simulink library "LPVBlockLibrary"  (R2014b)
settings: Solver=ode45  StartTime=0.0  StopTime=10.0  RelTol=1e-3
values from neighbouring files (symbols this model uses):
  ABMat = {Mab11, Mab12, Mab21, Mab22}    [lpvblkinit.m]
  CDMat = {Mcd11, Mcd12, Mcd21, Mcd22}    [lpvblkinit.m]
  dIVData = nan    [lpvblkinit.m]
  IVData = cell(numel(loc),1)    [lpvblkinit.m]
  LIVData = LIVData(loc)    [lpvblkinit.m]
  niv = numel(plist)    [lpvblkinit.m]
  nU = szS(2)    [lpvblkinit.m]
undefined symbols (not defined in the file or in its folder): x0
undefined symbols (not defined in the file): sys
libraries: LPVBlockLibrary x1
settings Model: Creator=musyn  LastModifiedBy=Arnar

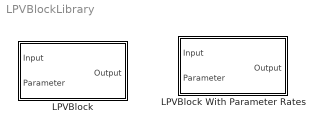
== system LPVBlockLibrary ==
  LPVBlock : Subsystem  mask{sys=sys, plist={'rho'}, x0=0}
      mask prompts: sys "System"; plist "ParameterVectorInputList (cell)"; x0 "Initial Condition"
      mask init:
      | [nU,ABMat,CDMat,IVData,dIVData,niv,LIVData] = ...
      |     lpvblkinit(sys,plist);
  LPVBlock With Parameter Rates : Subsystem  mask{sys=sys, plist={'rho'}, x0=x0, ratetc={'rho' 0.01}}
      mask prompts: sys "System"; plist "ParameterVectorInputList (cell)"; x0 "Initial Condition"; ratetc "Parameter Rate Time Constants"
      mask help:
      | Parameter Rate Time Constants:
      | N-by-2 cell array with each row being
      |    { char, time constant}.
      | The char specifies the parameter to be differentiated, e.g. 'rho'.
      | This parameter value will be approximately differentiated using
      | a high pass filter with the specified time constant.  The parameter
      | derivative must be an independent variable of the input PSS
      | specified in the form [char 'Dot'], e.g. 'rhoDot'.
      mask init:
      | if size(ratetc,2)~=2
      |     error('Parameter Rate Time Constants must be an N-by-2 cell array');
      | end
      | nrate = size(ratetc,1);
      | prate = ratetc(:,1);
      | nplist = length(plist);
      | 
      | [tfidx,prateidx] = ismember(prate,plist);
      | if all(tfidx)
      |     for i=1:nrate
      |         prate{i} = [prate{i} 'Dot'];
      |     end    
      |     pALL = [plist(:); prate(:)];
      | else
      |     % TODO PJS 5/28/2011: Improve error messages
      |     error('Parameters listed in rate time constants must be a subset of Parameter list');
      | end
      | 
      | % Convert to state space form
      | %   G(s) = s/(tau*s+1) = 1/tau
      | %
      | %   tau dx/dt +x = u
      | % --> dx/dt = -1/tau *x + 1/tau *u
      | tc = cell2mat(ratetc(:,2));
      | Ahp = diag( -1./tc );
      | Bhp = diag( -1./tc );
      | Chp = diag(  1./tc );
      | Dhp = diag(  1./tc );
      | 
      | % TODO PJS 5/28/2011: How should filter initial
      | % condition be handled?
      | xhp0 = zeros(nrate,1);

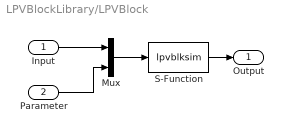
== system LPVBlockLibrary/LPVBlock ==
  Input : Inport
  Parameter : Inport  Port=2
  Mux : Mux  Inputs=[nU niv]
  S-Function : S-Function  FunctionName=lpvblksim  Parameters=nU,ABMat,CDMat,IVData,dIVData,niv,LIVData,x0  EnableBusSupport=off
  Output : Outport
  wires:
  Mux/1 -> S-Function/1
  Input/1 -> Mux/1
  S-Function/1 -> Output/1
  Parameter/1 -> Mux/2

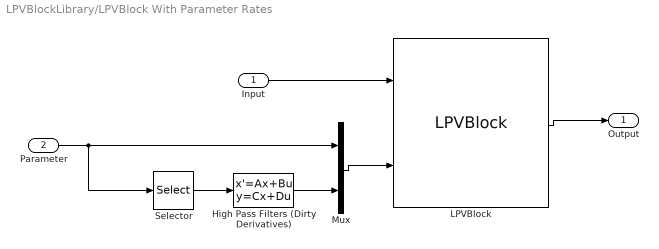
== system LPVBlockLibrary/LPVBlock With Parameter Rates ==
  Input : Inport
  Parameter : Inport  Port=2
  High Pass Filters (Dirty Derivatives) : StateSpace  A=Ahp  B=Bhp  C=Chp  D=Dhp  X0=zeros( size(Ahp,1), 1)
  LPVBlock : LPVBlockLibrary/LPVBlock  SystemSampleTime=-1  sys=sys  plist=pALL  x0=x0
  Mux : Mux  Inputs=2
  Selector : Selector  InputPortWidth=nplist  Indices=prateidx
  Output : Outport
  wires:
  Selector/1 -> High Pass Filters (Dirty Derivatives)/1
  High Pass Filters (Dirty Derivatives)/1 -> Mux/2
  LPVBlock/1 -> Output/1
  Parameter/1 -> Selector/1, Mux/1
  Mux/1 -> LPVBlock/2
  Input/1 -> LPVBlock/1
